simulink model "enablesub"  (Simulink 6.0)
settings: Solver=VariableStepDiscrete  StartTime=0.0  StopTime=10.0  RelTol=1e-3
settings Model: CovMetricSettings=d  Creator=The MathWorks Inc.  LastModifiedBy=batserve  ExtModeTrigMode=oneshot  ExtModeArmWhenConnect=off  ExtModeAutoUpdateStatusClock=off
settings DataIOCC: LimitDataPoints=off  SaveOutput=off  SaveTime=off
settings DebuggingCC: CheckExecutionContextPreStartOutputMsg=on  CheckExecutionContextRuntimeOutputMsg=on  SolverPrmCheckMsg=none  IntegerOverflowMsg=none
settings HardwareCC: TargetUnknown=on

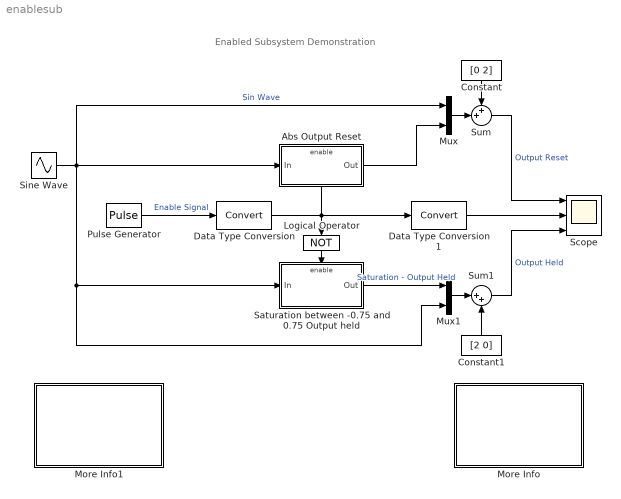
== system enablesub ==
  note: Enabled Subsystem Demonstration
  Abs Output Reset : Subsystem  TreatAsAtomicUnit=on  PropExecContextAcrossSSBoundary=on
  Constant : Constant  Orientation=down  Value=[0 2]
  Constant1 : Constant  Orientation=up  Value=[2 0]
  Data Type Conversion : DataTypeConversion  OutDataTypeMode=boolean  SaturateOnIntegerOverflow=on  RndMeth=Zero
  Data Type Conversion1 : DataTypeConversion  OutDataTypeMode=double  SaturateOnIntegerOverflow=on  RndMeth=Zero
  Logical Operator : Logic  Orientation=down  Operator=NOT  Inputs=1
  More Info : Subsystem  PropExecContextAcrossSSBoundary=on
      mask Display: disp('Double click\nhere for\ninformation on\nthis demonstration')
  More Info1 : Subsystem  PropExecContextAcrossSSBoundary=on
      settings: OpenFcn=simcad(bdroot);
      mask Display: disp('Double click\nhere for\nSimulink Help')
  Mux : Mux  Inputs=2
  Mux1 : Mux  Inputs=2
  Pulse Generator : DiscretePulseGenerator  PulseType=Time based  Period=5  PulseWidth=50
      settings: AttributesFormatString=Period: %<period>\nDuty cycle: %<pulsewidth>%
  Saturation between -0.75 and 0.75 Output held : Subsystem  TreatAsAtomicUnit=on  PropExecContextAcrossSSBoundary=on
  Scope : Scope  NumInputPorts=3
      settings: StartFcn=open_system(gcbh)  TickLabels=on  TimeRange=10  YMin=-1.6~-0.1~-1.5  YMax=3.6~1.1~3.5  DataFormat=Structure
  Sine Wave : Sin  SampleTime=0
  Sum : Sum  Inputs=++|  SaturateOnIntegerOverflow=on  InputSameDT=on
  Sum1 : Sum  Inputs=|++  SaturateOnIntegerOverflow=on  InputSameDT=on
  wires:
  Sine Wave/1 -> Abs Output Reset/1(In), Mux/1, Saturation between -0.75 and 0.75 Output held/1(In), Mux1/2  "Sin Wave"
  Saturation between -0.75 and 0.75 Output held/1(Out) -> Mux1/1  "Saturation - Output Held"
  Logical Operator/1 -> Saturation between -0.75 and 0.75 Output held/Enable
  Constant/1 -> Sum/1
  Mux/1 -> Sum/2
  Abs Output Reset/1(Out) -> Mux/2
  Sum/1 -> Scope/1  "Output Reset"
  Mux1/1 -> Sum1/1
  Constant1/1 -> Sum1/2
  Pulse Generator/1 -> Data Type Conversion/1  "Enable Signal"
  Sum1/1 -> Scope/3  "Output Held"
  Data Type Conversion/1 -> Logical Operator/1, Abs Output Reset/Enable, Data Type Conversion1/1
  Data Type Conversion1/1 -> Scope/2

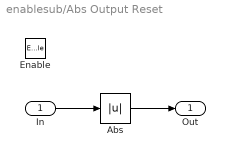
== system enablesub/Abs Output Reset ==
  In : Inport  Port=1  LatchInput=off
  Enable : EnablePort  StatesWhenEnabling=reset
  Abs : Abs  SaturateOnIntegerOverflow=on
  Out : Outport  OutputWhenDisabled=reset  InitialOutput=0
  wires:
  In/1 -> Abs/1
  Abs/1 -> Out/1

== system enablesub/More Info ==
  note: This demonstration shows what happens when a sign wave is fed into an
      | enabled subsystem.  After running the simulation, the scope shows three
      | plots.
      |
      | The first of these plots shows the original sine wave and the absolute
      | value of the original sine wave offset by two.  The absolute value of the sine
      | wave is only shown when the subsystem is enabled.  This occurs between
      | 0 and 2.5 seconds and 5 and 7.5 seconds.  When the subsystem is not
      | enabled then the output of the subsystem is reset to 0.  The value of 0 is
      | determined by the initial condition of the outport. You can see when
      | the subsysytem is enabled by looking at the second plot.  A value of 1
      | indicates that it is enabled.
      |
      | The second plot shows the original value of the enable signal.  If the signal
      | is towards the top of the plot then the subsystem related to the first plot
      | is enabled.  If the signal is towards the bottom of the plot then the
      | subsystem related to the third plot is enabled.  The difference on when the
      | subsystems are enabled is caused by the logical NOT block.
      |
      | The third plot shows the original sine wave and the saturation limited sine
      | wave offset by two.  The saturated value of the sine wave is only shown when
      | the subsystem is enabled.  This occurs between 2.5 and 5 seconds and 7.5
      | and 10 seconds.
  note: Enabled Subsystem Demonstration

== system enablesub/More Info1 ==

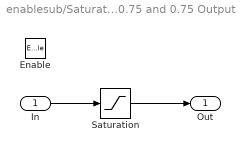
== system enablesub/Saturation between -0.75 and 0.75 Output held ==
  In : Inport  Port=1  LatchInput=off
  Enable : EnablePort
  Saturation : Saturate  UpperLimit=0.75  LowerLimit=-0.75
  Out : Outport
  wires:
  Saturation/1 -> Out/1
  In/1 -> Saturation/1
